simulink model "Ej_2"  (Simulink 8.7)
settings: Solver=ode3  StartTime=0.0  StopTime=100  FixedStep=0.0001  RelTol=1e-3
settings Model: Creator=Milton  LastModifiedBy=usuario
settings DataIOCC: SignalLoggingSaveFormat=ModelDataLogs
settings OptimizationCC: ExpressionDepthLimit=2147483647  EfficientMapNaN2IntZero=off
settings DebuggingCC: SolverPrmCheckMsg=warning  FcnCallInpInsideContextMsg=UseLocalSettings  AllowSymbolicDim=off  StateNameClashWarn=warning
settings HardwareCC: TargetBitPerPointer=64  TargetLongLongMode=on  TargetIntDivRoundTo=Zero  TargetEndianess=LittleEndian  TargetWordSize=64  TargetHWDeviceType=MATLAB Host  ProdEqTarget=off
settings RTWCC: SystemTargetFile=accel.tlc  TemplateMakefile=accel_default_tmf  RTWVerbose=off
settings CodeAppCC: MaxIdLength=128
settings STFCustomTargetCC: GeneratePreprocessorConditionals=Disable all  MATLABClassNameForMDSCustomization=Simulink.SoftwareTarget.TargetSpecificTriggerConfigurationBase  SystemTargetFile=accel.tlc

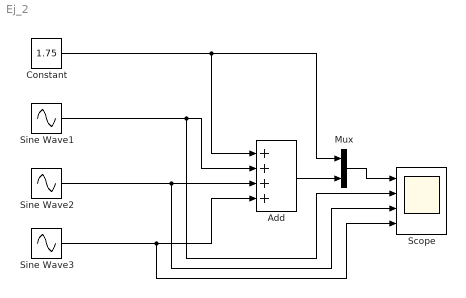
== system Ej_2 ==
  Add : Sum  Inputs=++++  RndMeth=Nearest
  Constant : Constant  Value=1.75  SampleTime=-1
  Mux : Mux  Inputs=2
  Scope : Scope  NumInputPorts=4
  Sine Wave1 : Sin  Amplitude=0.608  Frequency=2*pi*(pi/40)*1  Phase=pi/2
  Sine Wave2 : Sin  Amplitude=0.0675  Frequency=2*pi*3*(pi/40)  Phase=pi/2
  Sine Wave3 : Sin  Amplitude=0.0243  Frequency=2*pi*5*(pi/40)  Phase=pi/2
  wires:
  Constant/1 -> Add/1, Mux/1
  Sine Wave1/1 -> Add/2, Scope/2
  Sine Wave2/1 -> Add/3, Scope/3
  Sine Wave3/1 -> Add/4, Scope/4
  Add/1 -> Mux/2
  Mux/1 -> Scope/1
